simulink model "wecSimApps_converted"  (R2024a)
settings: Solver=ode4  StartTime=0  StopTime=3000  FixedStep=0.1  MaxStep=0.1  RelTol=1e-3  AbsTol=1e-3  EnableMultiTasking=on
values from neighbouring files (symbols this model uses):
  simu = simulationClass()    [wecSimInputFile.m]
undefined symbols (not defined in the file or in its folder): body, constraint, geometry, hydroData, pto, X, Y, Z
libraries: nesl_utility x22, fl_lib x20, SimscapeFluids_lib x10, sm_lib x6, WECSim_Lib_Constraints x4, WECSim_Lib_Body_Elements x2, WECSim_Lib_Frames x1, fl_ps_legacy_lib x1
(part 2 of 2)

== system wecSimApps_converted/Piston & RO   /Pressure Exchanger/Hydraulic Motor ==
  Hydraulic Motor : SimscapeFluids_lib/Isothermal Liquid/Pumps & Motors/Fixed-Displacement Motor (IL)  leakage_friction_spec=fluids.isothermal_liquid.pumps_motors.enum.MotorLossSpec.Analytical  displacement=5e-6 m^3/rad  omega_nominal=188 rad/s  p_nominal=100e5 Pa  vol_eff_nominal=1  mech_eff_nominal=1  no_load_torque=0 N*m  p_diff_eff_TLU=[100000.0, 1000000.0, 2000000.0] Pa  omega_eff_TLU=[25.0, 50.0, 100.0, 200.0, 300.0, 400.0] rad/s  vol_eff_TLU=[0.816, 0.908, 0.954, 0.977, 0.981, 0.984; 0.325, 0.663, 0.831, 0.916, 0.925, 0.946; 0.137, 0.568, 0.78, 0.892, 0.893, 0.91]  mech_eff_TLU=[0.996, 0.996, 0.996, 0.996, 0.996, 0.996; 0.988, 0.989, 0.989, 0.989, 0.989, 0.99; 0.981, 0.981, 0.982, 0.982, 0.983, 0.984]  p_diff_loss_TLU=[100000.0, 1000000.0, 2000000.0] Pa  omega_loss_TLU=[25.0, 50.0, 100.0, 200.0, 300.0, 400.0] rad/s  vol_loss_TLU=[0.0282, 0.0253, 0.0241, 0.0235, 0.0291, 0.0325; 0.2596, 0.1271, 0.1017, 0.0917, 0.1216, 0.1142; 0.7874, 0.1901, 0.141, 0.1211, 0.1797, 0.1978] * 1e-3 m^3/s  mech_loss_TLU=[0.002, 0.002, 0.002, 0.002, 0.002, 0.002; 0.06, 0.055, 0.055, 0.055, 0.055, 0.05; 0.19, 0.19, 0.18, 0.18, 0.17, 0.16] N*m  q_shaft_TLU=[.125, .25, .5, 1, 1.5, 2] * 1e-3 m^3/s  p_diff_shaft_TLU=[.1, 1, 2] MPa  torque_shaft_TLU=[.47, 4.72, 9.35; .47, 4.7, 9.36; .47, 4.7, 9.4; .47, 4.7, 9.41; .47, 4.7, 9.46; .47, 4.68, 9.5] N*m  omega_shaft_TLU=[205, 80, 35; 455, 330, 285; 955, 831, 780; 1950, 1830, 1780; 2940, 2775, 2680; 3940, 3780, 3640] rpm  vol_eff_min=1e-3  vol_eff_max=1  mech_eff_min=1e-3  mech_eff_max=1  pressure_threshold=1e5 Pa  omega_threshold=10 rad/s  supplied_range_check=simscape.enum.assert.action.none  motor_mode_check=simscape.enum.assert.action.none  pressure_check=simscape.enum.assert.action.none  p_min_valid=0 + 101325 Pa
      settings: LibrarySourceBlock=SimscapeFluids_lib/Isothermal Liquid/Pumps & Motors/Fixed-Displacement Motor (IL)  InternalSimscapePortConfiguration="{\"Bottom\":[{\"id\":\"B\",\"label\":\"B\",\"type\":\"foundation.isothermal_liquid.isothermal_liquid\"}],\"Left\":[],\"Right\":[{\"id\":\"R\",\"label\":\"R\",\"type\":\"foundation.mechanical.rotational.rotational\"},{\"id\":\"C\",\"label\":\"C\",\"type\":\"foundation.mechanical.rotational.rotational\"}],\"Top\":[{\"id\":\"A\",\"label\":\"A\",\"type\":\"foundation.isothermal_liquid.isothermal_liquid\"}]}"
  Mechanical Rotational Reference : fl_lib/Mechanical/Rotational Elements/Mechanical Rotational Reference
  A : PMIOPort  Side=Left
  S : PMIOPort  Port=2  Side=Right
  B : PMIOPort  Port=3  Side=Left
  connections:
  Hydraulic Motor/RConn3 -- B/RConn1
  Mechanical Rotational Reference/LConn1 -- Hydraulic Motor/RConn2
  S/RConn1 -- Hydraulic Motor/RConn1
  A/RConn1 -- Hydraulic Motor/LConn1

== system wecSimApps_converted/Piston & RO   /Pressure Exchanger/Hydraulic Flow Rate Sensor 1 ==
  Hydraulic Flow Rate Sensor 1 : fl_lib/Isothermal Liquid/Sensors/Flow Rate Sensor (IL)  sensor_type=3
      settings: LibrarySourceBlock=fl_lib/Isothermal Liquid/Sensors/Flow Rate Sensor (IL)  InternalSimscapePortConfiguration="{\"Bottom\":[],\"Left\":[{\"id\":\"A\",\"label\":\"A\",\"type\":\"foundation.isothermal_liquid.isothermal_liquid\"}],\"Right\":[{\"id\":\"B\",\"label\":\"B\",\"type\":\"foundation.isothermal_liquid.isothermal_liquid\"},{\"id\":\"M\",\"label\":\"M\",\"type\":\"output\"},{\"id\":\"V\",\"label\":\"V\",\"type\":\"output\"}],\"Top\":[]}"
  A : PMIOPort  Side=Left
  M : PMIOPort  Port=2  Side=Right
  V : PMIOPort  Port=3  Side=Right
  B : PMIOPort  Port=4  Side=Right
  connections:
  A/RConn1 -- Hydraulic Flow Rate Sensor 1/LConn1
  V/RConn1 -- Hydraulic Flow Rate Sensor 1/RConn3
  B/RConn1 -- Hydraulic Flow Rate Sensor 1/RConn1
  M/RConn1 -- Hydraulic Flow Rate Sensor 1/RConn2

== system wecSimApps_converted/Piston & RO   /Pressure Exchanger/Hydraulic Flow Rate Sensor 2 ==
  Hydraulic Flow Rate Sensor 2 : fl_lib/Isothermal Liquid/Sensors/Flow Rate Sensor (IL)  sensor_type=3
      settings: LibrarySourceBlock=fl_lib/Isothermal Liquid/Sensors/Flow Rate Sensor (IL)  InternalSimscapePortConfiguration="{\"Bottom\":[],\"Left\":[{\"id\":\"A\",\"label\":\"A\",\"type\":\"foundation.isothermal_liquid.isothermal_liquid\"}],\"Right\":[{\"id\":\"B\",\"label\":\"B\",\"type\":\"foundation.isothermal_liquid.isothermal_liquid\"},{\"id\":\"M\",\"label\":\"M\",\"type\":\"output\"},{\"id\":\"V\",\"label\":\"V\",\"type\":\"output\"}],\"Top\":[]}"
  B : PMIOPort  Side=Right
  M : PMIOPort  Port=2  Side=Right
  V : PMIOPort  Port=3  Side=Right
  A : PMIOPort  Port=4  Side=Left
  connections:
  Hydraulic Flow Rate Sensor 2/RConn2 -- M/RConn1
  B/RConn1 -- Hydraulic Flow Rate Sensor 2/RConn1
  A/RConn1 -- Hydraulic Flow Rate Sensor 2/LConn1
  V/RConn1 -- Hydraulic Flow Rate Sensor 2/RConn3

== system wecSimApps_converted/Piston & RO   /RO Membrane/Hydraulic Flow Rate Sensor 1 ==
  Hydraulic Flow Rate Sensor 1 : fl_lib/Isothermal Liquid/Sensors/Flow Rate Sensor (IL)  sensor_type=3
      settings: LibrarySourceBlock=fl_lib/Isothermal Liquid/Sensors/Flow Rate Sensor (IL)  InternalSimscapePortConfiguration="{\"Bottom\":[],\"Left\":[{\"id\":\"A\",\"label\":\"A\",\"type\":\"foundation.isothermal_liquid.isothermal_liquid\"}],\"Right\":[{\"id\":\"B\",\"label\":\"B\",\"type\":\"foundation.isothermal_liquid.isothermal_liquid\"},{\"id\":\"M\",\"label\":\"M\",\"type\":\"output\"},{\"id\":\"V\",\"label\":\"V\",\"type\":\"output\"}],\"Top\":[]}"
  V : PMIOPort  Side=Right
  A : PMIOPort  Port=2  Side=Left
  B : PMIOPort  Port=3  Side=Right
  M : PMIOPort  Port=4  Side=Right
  connections:
  Hydraulic Flow Rate Sensor 1/RConn3 -- V/RConn1
  Hydraulic Flow Rate Sensor 1/RConn1 -- B/RConn1
  Hydraulic Flow Rate Sensor 1/RConn2 -- M/RConn1
  A/RConn1 -- Hydraulic Flow Rate Sensor 1/LConn1

== system wecSimApps_converted/Piston & RO   /RO Membrane/Hydraulic Flow Rate Sensor 2 ==
  Hydraulic Flow Rate Sensor 2 : fl_lib/Isothermal Liquid/Sensors/Flow Rate Sensor (IL)  sensor_type=3
      settings: LibrarySourceBlock=fl_lib/Isothermal Liquid/Sensors/Flow Rate Sensor (IL)  InternalSimscapePortConfiguration="{\"Bottom\":[],\"Left\":[{\"id\":\"A\",\"label\":\"A\",\"type\":\"foundation.isothermal_liquid.isothermal_liquid\"}],\"Right\":[{\"id\":\"B\",\"label\":\"B\",\"type\":\"foundation.isothermal_liquid.isothermal_liquid\"},{\"id\":\"M\",\"label\":\"M\",\"type\":\"output\"},{\"id\":\"V\",\"label\":\"V\",\"type\":\"output\"}],\"Top\":[]}"
  V : PMIOPort  Side=Right
  A : PMIOPort  Port=2  Side=Left
  M : PMIOPort  Port=3  Side=Right
  B : PMIOPort  Port=4  Side=Right
  connections:
  Hydraulic Flow Rate Sensor 2/RConn2 -- M/RConn1
  Hydraulic Flow Rate Sensor 2/RConn1 -- B/RConn1
  Hydraulic Flow Rate Sensor 2/RConn3 -- V/RConn1
  A/RConn1 -- Hydraulic Flow Rate Sensor 2/LConn1
